simulink model "Athena_HIL_Test"  (R2024b)
settings: Solver=ode4  StartTime=0.0  StopTime=inf  FixedStep=0.001  RelTol=1e-3
undefined symbols (not defined in the file or in its folder): Payload
libraries: uavmavlinklib x3, dspnetwork x2, shared6dof x1
settings Model: Creator=ercu  LastModifiedBy=ercu

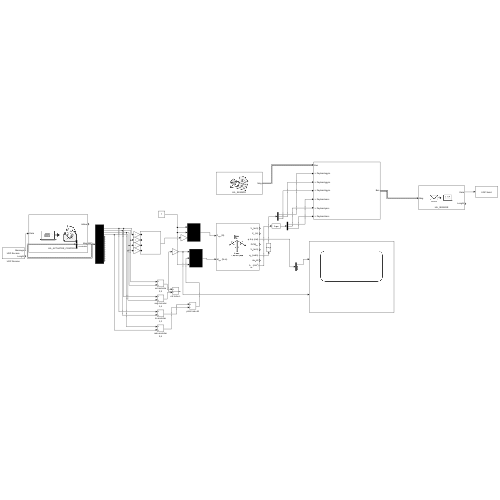
[thumbnail: Simulink's stored preview of the top-level diagram]
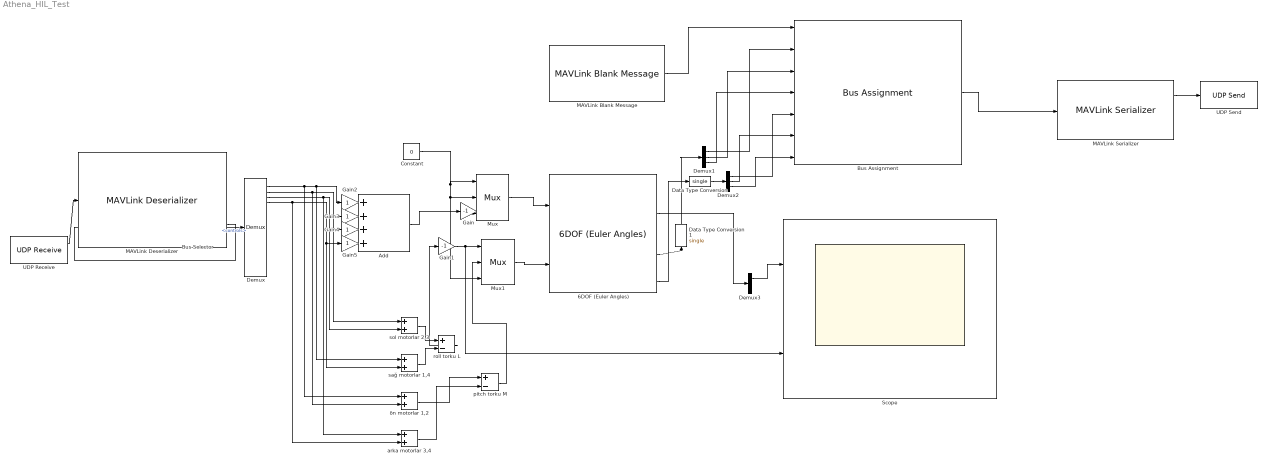
== system Athena_HIL_Test ==
  6DOF (Euler Angles) : shared6dof/6DOF (Euler Angles)  units=Metric (MKS)  mtype=Fixed  rep=Euler Angles  xme_0=[0 0 -10]  Vm_0=[0 0 0]  eul_0=[0.5 0 0]  pm_0=[0 0 0]  mass_0=1.0  mass_e=0.5  mass_f=2.0  inertia=eye(3) * 0.04  inertia_e=eye(3)  inertia_f=2*eye(3)  k_quat=1.0  vre_flag=on  abi_flag=off  aMode=0  xme_statename=''  Vm_statename=''  eul_statename=''  quat_statename=''  pm_statename=''  mass_statename=''
  Add : Sum  Inputs=++++  OutDataTypeStr=double
  Bus Assignment : BusAssignment  AssignedSignals=Payload.xgyro,Payload.ygyro,Payload.zgyro,Payload.xacc,Payload.yacc,Payload.zacc
  Bus Selector : BusSelector  OutputSignals=Payload.controls
  Constant : Constant  Value=0  OutDataTypeStr=double
  Data Type Conversion : DataTypeConversion  OutDataTypeStr=single  SaturateOnIntegerOverflow=off  RndMeth=Floor
  Data Type Conversion1 : DataTypeConversion  OutDataTypeStr=single  SaturateOnIntegerOverflow=off  RndMeth=Floor
  Demux : Demux  Outputs=16
  Demux1 : Demux  Outputs=3
  Demux2 : Demux  Outputs=3
  Demux3 : Demux  Outputs=3
  Gain : Gain  Gain=-1
  Gain1 : Gain  Gain=-1
  Gain{2..5} (4 alike) : Gain
  MAVLink Blank Message : uavmavlinklib/MAVLink Blank Message  dialectSource=Select from standard MAVLink dialects  dialect=common.xml  dialectCustom=common.xml  version=2  messageType=HIL_SENSOR  SystemID=1  ComponentID=1  SampleTime=inf
  MAVLink Deserializer : uavmavlinklib/MAVLink Deserializer  dialectSource=Select from standard MAVLink dialects  dialect=common.xml  dialectCustom=common.xml  version=2  messageType=HIL_ACTUATOR_CONTROLS  inputDataLength=off  SystemIDFilter=off  systemID=1  ComponentIDFilter=off  componentID=1  queueMsg=off  queueMsgSize=50  dropNum=off
  MAVLink Serializer : uavmavlinklib/MAVLink Serializer  dialectSource=Select from standard MAVLink dialects  dialect=common.xml  dialectCustom=common.xml  version=2  messageType=HIL_SENSOR
  Mux : Mux  Inputs=3
  Mux1 : Mux  Inputs=3
  Scope : Scope  NumInputPorts=2
  UDP Receive : dspnetwork/UDP Receive  localURL='0.0.0.0'  localPort=14550  remoteURL='127.0.0.1'  remotePort=-1  recvBufferSize=8192  dims=512  signalDatatype=uint8  isComplex=off  isVarSize=off  showBlockingTime=off  blockingTime=0  sampletime=0.004  blockPlatform=[]
      settings: LibrarySourceBlock=dspsrcs4/UDP Receive
  UDP Send : dspnetwork/UDP Send  remoteURL='127.0.0.1'  remotePort=14551  localURL='0.0.0.0'  localPortSource=Automatically determine  localPort=-1  sendBufferSize=8192  sampletime=-1  blockPlatform=[]  separateLengthPort=0
      settings: LibrarySourceBlock=dspsnks4/UDP Send
  arka motorlar 3,4 : Sum
  pitch torku M : Sum  Inputs=+-  OutDataTypeStr=double
  roll torku L : Sum  Inputs=+-  OutDataTypeStr=double
  sağ motorlar 1,4 : Sum
  sol motorlar 2,3 : Sum
  ön motorlar 1,2 : Sum
  wires:
  MAVLink Serializer/1 -> UDP Send/1
  UDP Receive/1 -> MAVLink Deserializer/1
  MAVLink Blank Message/1 -> Bus Assignment/1
  Bus Assignment/1 -> MAVLink Serializer/1
  MAVLink Deserializer/2 -> Bus Selector/1
  Bus Selector/1 -> Demux/1  "<controls>"
  Demux/1 -> ön motorlar 1,2/1, sağ motorlar 1,4/1, Gain2/1
  Demux/2 -> ön motorlar 1,2/2, sol motorlar 2,3/1, Gain3/1
  Demux/3 -> arka motorlar 3,4/1, sol motorlar 2,3/2, Gain4/1
  Demux/4 -> arka motorlar 3,4/2, sağ motorlar 1,4/2, Gain5/1
  Add/1 -> Gain/1
  Constant/1 -> Mux1/3, Mux/2, Mux/1
  Mux/1 -> 6DOF (Euler Angles)/1
  Mux1/1 -> 6DOF (Euler Angles)/2
  sol motorlar 2,3/1 -> roll torku L/1
  sağ motorlar 1,4/1 -> roll torku L/2
  ön motorlar 1,2/1 -> pitch torku M/1
  arka motorlar 3,4/1 -> pitch torku M/2
  pitch torku M/1 -> Mux1/2
  6DOF (Euler Angles)/6 -> Data Type Conversion1/1
  Demux1/1 -> Bus Assignment/2
  Demux1/2 -> Bus Assignment/3
  Demux1/3 -> Bus Assignment/4
  6DOF (Euler Angles)/8 -> Data Type Conversion/1
  Demux2/1 -> Bus Assignment/5
  Demux2/2 -> Bus Assignment/6
  Demux2/3 -> Bus Assignment/7
  6DOF (Euler Angles)/3 -> Demux3/1
  Demux3/1 -> Scope/1
  Data Type Conversion/1 -> Demux2/1
  Data Type Conversion1/1 -> Demux1/1
  Gain/1 -> Mux/3
  roll torku L/1 -> Gain1/1
  Gain1/1 -> Scope/2, Mux1/1
  Gain2/1 -> Add/1
  Gain3/1 -> Add/2
  Gain5/1 -> Add/4
  Gain4/1 -> Add/3
